simulink model "HANcoder_E407_GTSync_v5"  (R2018b)
settings: Solver=FixedStepDiscrete  StartTime=0.0  StopTime=1  FixedStep=0.01  RelTol=1e-3
PreLoadFcn:
  | librarySetup
  | eval([bdroot,'_startup']) %Calling [modelName]_startup.m
values from neighbouring files (symbols this model uses):
  basic_cycle_duration = TM_Reset_Board + COMP_duration    (= 170)    [HANcoder_E407_GTSync_v5_startup.m]
  comm_delay_estimation1 = round(comm_delay_measured*hardware_granularity/frequency_IRQ)    [HANcoder_E407_GTSync_v5_startup.m]
  comm_delay_estimation2 = round(comm_delay_measured*hardware_granularity/frequency_IRQ)    [HANcoder_E407_GTSync_v5_startup.m]
  COMM_Period = 25    [HANcoder_E407_GTSync_v5_startup.m]
  COMM_Phase1 = floor(COMM_Period/5)    [HANcoder_E407_GTSync_v5_startup.m]
  COMM_Phase2 = floor(4*COMM_Period/5)    [HANcoder_E407_GTSync_v5_startup.m]
  frequency_IRQ = 100    [HANcoder_E407_GTSync_v5_startup.m]
  HANtuneOverride = Simulink.Parameter    [HANcoder_E407_GTSync_v5_startup.m]
  idle_time_init = basic_cycle_duration*matrix_rows    (= 340)    [HANcoder_E407_GTSync_v5_startup.m]
  LED_ticks_toggle = 10000    [HANcoder_E407_GTSync_v5_startup.m]
  Master_Role = 1    [HANcoder_E407_GTSync_v5_startup.m]
  matrix_rows = 2    [HANcoder_E407_GTSync_v5_startup.m]
  MEX_Flag = 0    [HANcoder_E407_GTSync_v5_startup.m]
  Slave_Role = 2    [HANcoder_E407_GTSync_v5_startup.m]
  Sync_ID = 1    [HANcoder_E407_GTSync_v5_startup.m]
  TM_Check_Sync = TM_COMM_Sync   + COMM_duration    (= 30)    [HANcoder_E407_GTSync_v5_startup.m]
  TM_Check_TOuts = TM_Count_Vote3 + COMP_duration    (= 150)    [HANcoder_E407_GTSync_v5_startup.m]
  TM_Check_Vote1 = TM_COMM_Vote1  + COMM_duration    (= 70)    [HANcoder_E407_GTSync_v5_startup.m]
  TM_Check_Vote2 = TM_COMM_Vote2  + COMM_duration    (= 105)    [HANcoder_E407_GTSync_v5_startup.m]
  TM_Check_Vote3 = TM_COMM_Vote3  + COMM_duration    (= 140)    [HANcoder_E407_GTSync_v5_startup.m]
  TM_COMM_Sync = basic_cycle_start    (= 5)    [HANcoder_E407_GTSync_v5_startup.m]
  TM_COMM_Vote1 = TM_Vote_Dec    + COMP_duration    (= 45)    [HANcoder_E407_GTSync_v5_startup.m]
  TM_COMM_Vote2 = TM_Count_Vote1 + COMP_duration    (= 80)    [HANcoder_E407_GTSync_v5_startup.m]
  TM_COMM_Vote3 = TM_Count_Vote2 + COMP_duration    (= 115)    [HANcoder_E407_GTSync_v5_startup.m]
  TM_Count_Vote1 = TM_Check_Vote1 + COMP_duration    (= 75)    [HANcoder_E407_GTSync_v5_startup.m]
  TM_Count_Vote2 = TM_Check_Vote2 + COMP_duration    (= 110)    [HANcoder_E407_GTSync_v5_startup.m]
  TM_Count_Vote3 = TM_Check_Vote3 + COMP_duration    (= 145)    [HANcoder_E407_GTSync_v5_startup.m]
  TM_New_Master = TM_Check_TOuts + COMP_duration    (= 155)    [HANcoder_E407_GTSync_v5_startup.m]
  TM_Reset_Board = TM_Reset_Var   + COMP_duration    (= 165)    [HANcoder_E407_GTSync_v5_startup.m]
  TM_Reset_Var = TM_New_Master  + COMP_duration    (= 160)    [HANcoder_E407_GTSync_v5_startup.m]
  TM_Update_LT = TM_Check_Sync  + COMP_duration    (= 35)    [HANcoder_E407_GTSync_v5_startup.m]
  TM_Vote_Dec = TM_Update_LT   + COMP_duration    (= 40)    [HANcoder_E407_GTSync_v5_startup.m]
  Toggle_Flag = 1    [HANcoder_E407_GTSync_v5_startup.m]
  Vote1_ID = 12    [HANcoder_E407_GTSync_v5_startup.m]
  Vote2_ID = 22    [HANcoder_E407_GTSync_v5_startup.m]
  Vote3_ID = 32    [HANcoder_E407_GTSync_v5_startup.m]
undefined symbols (not defined in the file or in its folder): A0, A1, A2, A3, CON2
libraries: HANcoder_STM32_Target x25, hdlsllib x21, simulink x3, simulink_extras x1
(part 2 of 7)

== system HANcoder_E407_GTSync_v5/HANcoder STM32 Target - E407-STM32 algorithm/Global Ticks Increment/If Action Subsystem ==
  note: CAN ID Init
  Action Port : ActionPort  ActionType=then
  Add : Sum  Inputs=++++
  Constant : Constant
  Constant1 : Constant  Value=2
  Constant2 : Constant  Value=4
  Constant3 : Constant  Value=8
  Digital Input : HANcoder_STM32_Target/STM32-E407/Digital Inputs/Digital Input  Tag=HANcoder_TARGET_STM32_E407  pinID=CON3 - D2 - 5V Tolerant  config=Pulldown  tsamp=-1
      settings: SourceProductName=HANcoder STM32 Target
  Digital Input1 : HANcoder_STM32_Target/STM32-E407/Digital Inputs/Digital Input  Tag=HANcoder_TARGET_STM32_E407  pinID=CON3 - D3 - 5V Tolerant  config=Pulldown  tsamp=-1
      settings: SourceProductName=HANcoder STM32 Target
  Digital Input2 : HANcoder_STM32_Target/STM32-E407/Digital Inputs/Digital Input  Tag=HANcoder_TARGET_STM32_E407  pinID=CON3 - D4 - 5V Tolerant  config=Pulldown  tsamp=-1
      settings: SourceProductName=HANcoder STM32 Target
  Digital Input3 : HANcoder_STM32_Target/STM32-E407/Digital Inputs/Digital Input  Tag=HANcoder_TARGET_STM32_E407  pinID=CON3 - D5 - 5V Tolerant  config=Pulldown  tsamp=-1
      settings: SourceProductName=HANcoder STM32 Target
  Multiply{,1..3} (4 alike) : Product
  Out1 : Outport
  wires:
  Constant1/1 -> Multiply1/1
  Add/1 -> Out1/1
  Constant3/1 -> Multiply3/1
  Constant2/1 -> Multiply2/1
  Multiply2/1 -> Add/3
  Digital Input3/1 -> Multiply3/2
  Digital Input1/1 -> Multiply1/2
  Multiply3/1 -> Add/4
  Multiply1/1 -> Add/2
  Digital Input2/1 -> Multiply2/2
  Multiply/1 -> Add/1
  Digital Input/1 -> Multiply/2
  Constant/1 -> Multiply/1

== system HANcoder_E407_GTSync_v5/HANcoder STM32 Target - E407-STM32 algorithm/Global Ticks Increment/Initialize Clock Schedule ==
  Enable : EnablePort
  Constant : Constant  OutDataTypeStr=uint16
  Constant1 : Constant  Value=3  OutDataTypeStr=uint8
  Constant2 : Constant
  Data Store Write : DataStoreWrite  DataStoreName=init_clock
  Schedule Compare Event1 : HANcoder_STM32_Target/STM32-E407/Timer Outputs/Schedule Compare Event  Tag=HANcoder_TARGET_STM32_E407  pin=TIM4 - CON PD - 15 - 5V Tolerant  tsamp=-1
      settings: SourceProductName=HANcoder STM32 Target
  wires:
  Constant/1 -> Schedule Compare Event1/1
  Constant1/1 -> Schedule Compare Event1/2
  Constant2/1 -> Data Store Write/1

== system HANcoder_E407_GTSync_v5/HANcoder STM32 Target - E407-STM32 algorithm/Global Ticks Increment/Local Time generation ==
  note: Reschedule IRQ activation
  Clock_State : Inport
  function : TriggerPort  TriggerType=function-call  VariantControl=Variant
  Chart : Stateflow chart  TreatAsAtomicUnit=on
  Constant : Constant  Value=frequency_IRQ  OutDataTypeStr=uint16
  Constant1 : Constant  Value=3  OutDataTypeStr=uint8
  Constant2 : Constant  OutDataTypeStr=uint16
  Data Store Read : DataStoreRead  DataStoreName=Local_Ticks
  Data Store Read1 : DataStoreRead  DataStoreName=Local_Ticks
  Data Store Write : DataStoreWrite  DataStoreName=Local_Ticks
  Get Last Event Counter1 : HANcoder_STM32_Target/STM32-E407/Timer Outputs/Get Last Event Counter  Tag=HANcoder_TARGET_STM32_E407  pin=TIM4 - CON PD - 15 - 5V Tolerant  tsamp=-1
      settings: SourceProductName=HANcoder STM32 Target
  Schedule Compare Event : HANcoder_STM32_Target/STM32-E407/Timer Outputs/Schedule Compare Event  Tag=HANcoder_TARGET_STM32_E407  pin=TIM4 - CON PD - 15 - 5V Tolerant  tsamp=-1
      settings: SourceProductName=HANcoder STM32 Target
  Sum : Sum
  Sum1 : Sum
  Switch : Switch  Criteria=u2 > Threshold
  activate_CAN_management : Outport
  wires:
  Get Last Event Counter1/1 -> Sum/1
  Constant/1 -> Sum/2
  Sum/1 -> Schedule Compare Event/1
  Constant1/1 -> Schedule Compare Event/2
  Data Store Read1/1 -> Switch/3
  Data Store Read/1 -> Sum1/1
  Constant2/1 -> Sum1/2
  Clock_State/1 -> Chart/1(Condition), Switch/2
  Switch/1 -> Data Store Write/1  "local_ticks_interrupt"
  Sum1/1 -> Switch/1
  Chart/1(Trigger_Signal()) -> activate_CAN_management/1

== system HANcoder_E407_GTSync_v5/HANcoder STM32 Target - E407-STM32 algorithm/Global Ticks Increment/Measure EXecution time ==
  note: Measured Execution Time
  Trigger : TriggerPort  TriggerType=function-call  VariantControl=Variant
  Constant1 : Constant  Priority=1  Value=MEX_Flag
  DEBUG - Toggle digital pin A3 : Subsystem  Priority=3
  Data Store Memory4 : DataStoreMemory  DataStoreName=A3_Pin_State  ReadBeforeWriteMsg=warning  WriteAfterWriteMsg=warning  WriteAfterReadMsg=warning  ShowAdditionalParam=off  OutDataTypeStr=boolean
  wires:
  Constant1/1 -> DEBUG - Toggle digital pin A3/Enable

== system HANcoder_E407_GTSync_v5/HANcoder STM32 Target - E407-STM32 algorithm/Global Ticks Increment/Output Compare Init2 ==
  S-Function : S-Function  FunctionName=sfcn_timeout_init  SFunctionDeploymentMode=off  EnableBusSupport=off
  Term1 : Terminator
  wires:
  S-Function/1 -> Term1/1

== system HANcoder_E407_GTSync_v5/HANcoder STM32 Target - E407-STM32 algorithm/Operation Mode/Flip Flop T ==
  T : Inport  OutDataTypeStr=boolean
  Clk : Inport  Port=2  OutDataTypeStr=boolean
  J-K Flip-Flop : simulink_extras/Flip Flops/J-K Flip-Flop  initial_condition=0
      settings: SourceProductName=Simulink
  Terminator : Terminator
  Q : Outport  OutDataTypeStr=boolean
  wires:
  J-K Flip-Flop/2 -> Terminator/1
  T/1 -> J-K Flip-Flop/3, J-K Flip-Flop/1
  J-K Flip-Flop/1 -> Q/1
  Clk/1 -> J-K Flip-Flop/2

== system HANcoder_E407_GTSync_v5/HANcoder STM32 Target - E407-STM32 algorithm/Global Ticks Increment/CAN Management/Basic Cycle Increment ==
  note: Local Time Reset
  note: Basic cycle counter
  Enable : EnablePort
  Add : Sum
  Add1 : Sum  Inputs=+-
  Constant : Constant  Value=matrix_rows
  Data Store Read4 : DataStoreRead  DataStoreName=basic_cycle_count
  Data Store Read5 : DataStoreRead  DataStoreName=basic_cycle_count
  Data Store Write : DataStoreWrite  DataStoreName=Local_Ticks
  Data Store Write3 : DataStoreWrite  DataStoreName=basic_cycle_count
  Decrement : Constant  OutDataTypeStr=uint8
  Increment : Constant  OutDataTypeStr=uint8
  LessThanOrEqual : RelationalOperator  Operator=<  OutDataTypeStr=boolean  RndMeth=Simplest
  Reset : Constant  Value=0  OutDataTypeStr=uint16
  Switch : Switch  Criteria=u2 > Threshold
  wires:
  Switch/1 -> Data Store Write3/1  "bc"
  Data Store Read5/1 -> LessThanOrEqual/1
  Add/1 -> Switch/1
  Increment/1 -> Add/2
  Data Store Read4/1 -> Add/1
  LessThanOrEqual/1 -> Switch/2
  Constant/1 -> Add1/1
  Reset/1 -> Switch/3, Data Store Write/1
  Decrement/1 -> Add1/2
  Add1/1 -> LessThanOrEqual/2

== system HANcoder_E407_GTSync_v5/HANcoder STM32 Target - E407-STM32 algorithm/Global Ticks Increment/CAN Management/DEBUG - Toggle digital pin A0 ==
  note: Change pin state
  note: Reset condition
  note: Toggle pin data stored
  Enable : EnablePort
  Constant : Constant  OutDataTypeStr=boolean
  Constant1 : Constant  Value=0  OutDataTypeStr=boolean
  Constant2 : Constant  Value=0  OutDataTypeStr=boolean
  Data Store Read : DataStoreRead  DataStoreName=A0_Pin_State
  Data Store Read1 : DataStoreRead  DataStoreName=A0_Pin_State
  Data Store Write : DataStoreWrite  DataStoreName=Toggle_Pin_A0
  Data Store Write1 : DataStoreWrite  DataStoreName=A0_Pin_State
  Digital Output : HANcoder_STM32_Target/STM32-E407/Digital Outputs/Digital Output  Tag=HANcoder_TARGET_STM32_E407  pinID=CON2 - A0  config=Open drain  tsamp=-1
      settings: SourceProductName=HANcoder STM32 Target
  Switch : Switch  Criteria=u2 > Threshold
  wires:
  Switch/1 -> Data Store Write1/1
  Data Store Read/1 -> Switch/2
  Constant/1 -> Switch/3
  Constant1/1 -> Switch/1
  Constant2/1 -> Data Store Write/1
  Data Store Read1/1 -> Digital Output/1

== system HANcoder_E407_GTSync_v5/HANcoder STM32 Target - E407-STM32 algorithm/Global Ticks Increment/CAN Management/DEBUG - Toggle digital pin A1 ==
  note: Toggle pin data stored
  note: Reset condition
  note: Change pin state
  Enable : EnablePort
  Constant : Constant  OutDataTypeStr=boolean
  Constant1 : Constant  Value=0  OutDataTypeStr=boolean
  Constant2 : Constant  Value=0  OutDataTypeStr=boolean
  Data Store Read : DataStoreRead  DataStoreName=A1_Pin_State
  Data Store Read1 : DataStoreRead  DataStoreName=A1_Pin_State
  Data Store Write : DataStoreWrite  DataStoreName=Toggle_Pin_A1
  Data Store Write1 : DataStoreWrite  DataStoreName=A1_Pin_State
  Digital Output : HANcoder_STM32_Target/STM32-E407/Digital Outputs/Digital Output  Tag=HANcoder_TARGET_STM32_E407  pinID=CON2 - A1  config=Open drain  tsamp=-1
      settings: SourceProductName=HANcoder STM32 Target
  Switch : Switch  Criteria=u2 > Threshold
  wires:
  Data Store Read1/1 -> Digital Output/1
  Constant2/1 -> Data Store Write/1
  Constant1/1 -> Switch/1
  Constant/1 -> Switch/3
  Data Store Read/1 -> Switch/2
  Switch/1 -> Data Store Write1/1

== system HANcoder_E407_GTSync_v5/HANcoder STM32 Target - E407-STM32 algorithm/Global Ticks Increment/CAN Management/DEBUG - Toggle digital pin A2 ==
  note: Toggle pin data stored
  note: Change pin state
  Enable : EnablePort
  Constant : Constant  OutDataTypeStr=boolean
  Constant1 : Constant  Value=0  OutDataTypeStr=boolean
  Data Store Read : DataStoreRead  DataStoreName=A2_Pin_State
  Data Store Read1 : DataStoreRead  DataStoreName=A2_Pin_State
  Data Store Write1 : DataStoreWrite  DataStoreName=A2_Pin_State
  Digital Output : HANcoder_STM32_Target/STM32-E407/Digital Outputs/Digital Output  Tag=HANcoder_TARGET_STM32_E407  pinID=CON2 - A2  config=Open drain  tsamp=-1
      settings: SourceProductName=HANcoder STM32 Target
  Switch : Switch  Criteria=u2 > Threshold
  wires:
  Data Store Read1/1 -> Digital Output/1
  Constant1/1 -> Switch/1
  Constant/1 -> Switch/3
  Data Store Read/1 -> Switch/2
  Switch/1 -> Data Store Write1/1

== system HANcoder_E407_GTSync_v5/HANcoder STM32 Target - E407-STM32 algorithm/Global Ticks Increment/CAN Management/Initialization ==
  Enable : EnablePort  PropagateVarSize=During execution
  AND : Logic  IconShape=distinctive  AllPortsSameDT=off  OutDataTypeStr=boolean
  Board nr1 : Constant
  Constant : Constant  Value=idle_time_init
  Data Store Memory : DataStoreMemory  DataStoreName=Initialization_Timeout  ReadBeforeWriteMsg=warning  WriteAfterWriteMsg=warning  WriteAfterReadMsg=warning  ShowAdditionalParam=off  OutDataTypeStr=boolean
  Data Store Memory1 : DataStoreMemory  DataStoreName=Delay_Counter  ReadBeforeWriteMsg=warning  WriteAfterWriteMsg=warning  WriteAfterReadMsg=warning  ShowAdditionalParam=off  OutDataTypeStr=double
  Data Store Read : DataStoreRead  DataStoreName=New_Msg_Ready_CAN1
  Data Store Read1 : DataStoreRead  DataStoreName=Initialization_Timeout
  Data Store Read2 : DataStoreRead  DataStoreName=New_Msg_Ready_CAN2
  Data Store Read4 : DataStoreRead  DataStoreName=Board_ID
  Data Store Write : DataStoreWrite  DataStoreName=Initialization_Timeout
  Data Store Write1 : DataStoreWrite  DataStoreName=Initialization_flag
  Delay : Subsystem
  Equal : RelationalOperator  Operator===  OutDataTypeStr=boolean  RndMeth=Simplest
  NOT : Logic  Operator=NOT  IconShape=distinctive  AllPortsSameDT=off  OutDataTypeStr=boolean
  OR : Logic  Operator=OR  IconShape=distinctive  AllPortsSameDT=off  OutDataTypeStr=boolean
  OR1 : Logic  Operator=OR  IconShape=distinctive  AllPortsSameDT=off  OutDataTypeStr=boolean
  RoleID and Global Time init : Subsystem  TreatAsAtomicUnit=on
  wires:
  Delay/1(Output) -> Data Store Write/1
  Constant/1 -> Delay/1(Input)
  NOT/1 -> Data Store Write1/1
  RoleID and Global Time init/1(Finish Initialization) -> NOT/1
  OR/1 -> RoleID and Global Time init/Enable
  Data Store Read1/1 -> AND/2, RoleID and Global Time init/1(Timeout Initialization)
  OR1/1 -> OR/2, RoleID and Global Time init/2(Reference message received)
  Data Store Read4/1 -> Equal/1
  Board nr1/1 -> Equal/2
  Equal/1 -> AND/1
  AND/1 -> OR/1
  Data Store Read/1 -> OR1/1
  Data Store Read2/1 -> OR1/2

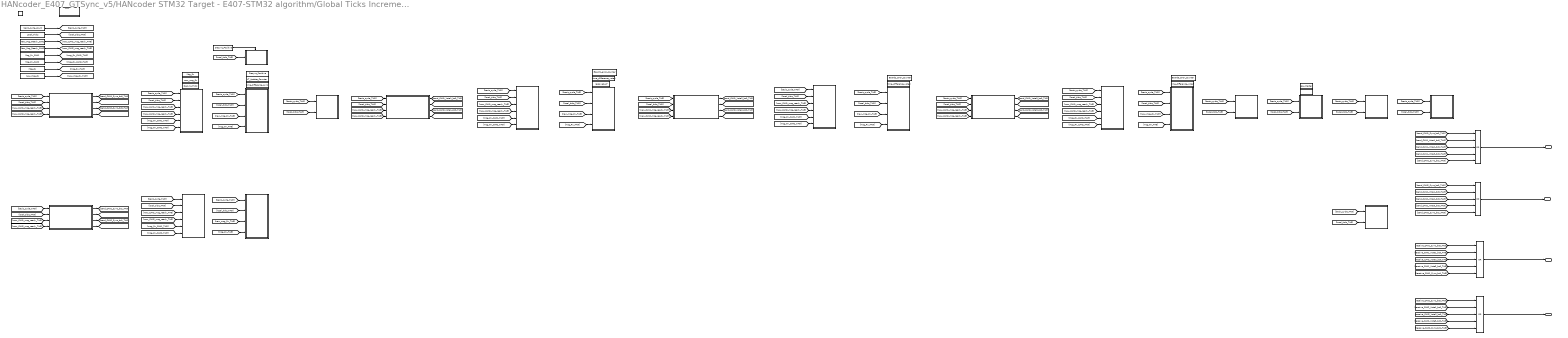
== system HANcoder_E407_GTSync_v5/HANcoder STM32 Target - E407-STM32 algorithm/Global Ticks Increment/CAN Management/Matrix Cycle Manager ==
  note: Receive message condition
      | Sync Msg: Not Master and TM0
      | Vote Msg: Not # Node at TM#
  note: Shortcut Tags
  note: Output Send_Message
      | Send: 1
      | Do not send: 0
  note: Send message condition
      | Sync Msg: Master and TM0
      | Vote Msg: Node# and TM#
  note: Output Receive_Message
      | Receive: 1
      | Do not receive: 0
  note: Receive message condition
      | Sync Msg: Not Master and TM0
      | Vote Msg: Not # Node at TM#
  note: Output Receive_Message
      | Receive: 1
      | Do not receive: 0
  note: Send message condition
      | Sync Msg: Master and TM0
      | Vote Msg: Node# and TM#
  note: Output Send_Message
      | Send: 1
      | Do not send: 0
  Enable : EnablePort  PropagateVarSize=During execution
  COMM Task - Sync BC0 : Subsystem
  COMM Task - Sync BC1 : Subsystem
  COMM Task - Vote1 : Subsystem
  COMM Task - Vote2 : Subsystem
  COMM Task - Vote3 : Subsystem
  COMP Task - Check Timeouts : Subsystem
  COMP Task - New Master : Subsystem
  COMP Task - Reset Board : Subsystem
  COMP Task - Reset Variables BC0 : Subsystem
  COMP Task - Reset Variables BC1 : Subsystem
  COMP Task - Rx_Sync_Check : Subsystem
  COMP Task - Rx_Sync_Check - bc1 : Subsystem
  COMP Task - Rx_Vote1_Check : Subsystem
  COMP Task - Rx_Vote2_Check : Subsystem
  COMP Task - Rx_Vote3_Check : Subsystem
  COMP Task - Update LT : Subsystem
  COMP Task - Update LT - bc1 : Subsystem
  COMP Task - Vote Decision : Subsystem
  COMP Task - Vote1 Count : Subsystem
  COMP Task - Vote2 Count : Subsystem
  COMP Task - Vote3 Count : Subsystem
  Data Store Memory : DataStoreMemory  DataStoreName=time_difference_sync  ReadBeforeWriteMsg=warning  WriteAfterWriteMsg=warning  WriteAfterReadMsg=warning  ShowAdditionalParam=off
  Data Store Memory1 : DataStoreMemory  DataStoreName=Board1_error_counter  ReadBeforeWriteMsg=warning  WriteAfterWriteMsg=warning  WriteAfterReadMsg=warning  ShowAdditionalParam=off  OutMin=0  OutMax=4294967294  OutDataTypeStr=double
  Data Store Memory10 : DataStoreMemory  DataStoreName=New_Master  ReadBeforeWriteMsg=warning  WriteAfterWriteMsg=warning  WriteAfterReadMsg=warning  ShowAdditionalParam=off  OutDataTypeStr=boolean
  Data Store Memory11 : DataStoreMemory  DataStoreName=Msg_Rx  ReadBeforeWriteMsg=warning  WriteAfterWriteMsg=warning  WriteAfterReadMsg=warning  ShowAdditionalParam=off  OutDataTypeStr=Bus: demux_msg_buffer_type
  Data Store Memory12 : DataStoreMemory  DataStoreName=LT_Update_Counter  ReadBeforeWriteMsg=warning  WriteAfterWriteMsg=warning  WriteAfterReadMsg=warning  ShowAdditionalParam=off
  Data Store Memory13 : DataStoreMemory  DataStoreName=Desync_Ticks  ReadBeforeWriteMsg=warning  WriteAfterWriteMsg=warning  WriteAfterReadMsg=warning  ShowAdditionalParam=off  OutDataTypeStr=double
  Data Store Memory14 : DataStoreMemory  DataStoreName=Desync_Positive  ReadBeforeWriteMsg=warning  WriteAfterWriteMsg=warning  WriteAfterReadMsg=warning  ShowAdditionalParam=off  OutDataTypeStr=boolean
  Data Store Memory2 : DataStoreMemory  DataStoreName=Board2_error_counter  ReadBeforeWriteMsg=warning  WriteAfterWriteMsg=warning  WriteAfterReadMsg=warning  ShowAdditionalParam=off  OutMin=0  OutMax=4294967294  OutDataTypeStr=double
  Data Store Memory3 : DataStoreMemory  DataStoreName=Board3_error_counter  ReadBeforeWriteMsg=warning  WriteAfterWriteMsg=warning  WriteAfterReadMsg=warning  ShowAdditionalParam=off  OutMin=0  OutMax=4294967294  OutDataTypeStr=double
  Data Store Memory4 : DataStoreMemory  DataStoreName=time_difference_vote1  ReadBeforeWriteMsg=warning  WriteAfterWriteMsg=warning  WriteAfterReadMsg=warning  ShowAdditionalParam=off
  Data Store Memory5 : DataStoreMemory  DataStoreName=time_difference_vote2  ReadBeforeWriteMsg=warning  WriteAfterWriteMsg=warning  WriteAfterReadMsg=warning  ShowAdditionalParam=off
  Data Store Memory6 : DataStoreMemory  DataStoreName=time_difference_vote3  ReadBeforeWriteMsg=warning  WriteAfterWriteMsg=warning  WriteAfterReadMsg=warning  ShowAdditionalParam=off
  Data Store Memory7 : DataStoreMemory  DataStoreName=Reset_Board  ReadBeforeWriteMsg=warning  WriteAfterWriteMsg=warning  WriteAfterReadMsg=warning  ShowAdditionalParam=off  OutDataTypeStr=boolean
  Data Store Memory8 : DataStoreMemory  DataStoreName=new_msg_Rx  ReadBeforeWriteMsg=warning  WriteAfterWriteMsg=warning  WriteAfterReadMsg=warning  ShowAdditionalParam=off
  Data Store Memory9 : DataStoreMemory  DataStoreName=received_LT  ReadBeforeWriteMsg=warning  WriteAfterWriteMsg=warning  WriteAfterReadMsg=warning  ShowAdditionalParam=off  OutDataTypeStr=Bus: received_vote_local_time
  Data Store Read : DataStoreRead  DataStoreName=Msg_Rx_CAN1
  Data Store Read1 : DataStoreRead  DataStoreName=New_Msg_Ready_CAN1
  Data Store Read10 : DataStoreRead  DataStoreName=basic_cycle_count
  Data Store Read2 : DataStoreRead  DataStoreName=New_Msg_Ready_CAN2
  Data Store Read3 : DataStoreRead  DataStoreName=Msg_Rx_CAN2
  Data Store Read4 : DataStoreRead  DataStoreName=Msg_Rx
  Data Store Read5 : DataStoreRead  DataStoreName=new_msg_Rx
  Data Store Read6 : DataStoreRead  DataStoreName=Desync_Positive
  Data Store Read9 : DataStoreRead  DataStoreName=Local_Ticks
  LT_Update Desync_Positive : Subsystem  Priority=100  TreatAsAtomicUnit=on
  Matrix_Cycle_Observation_DEBUG : Subsystem
  OR{1..4} (4 alike) : Logic  Operator=OR  Inputs=5  IconShape=distinctive  AllPortsSameDT=off  OutDataTypeStr=boolean
  Send_Message_CAN1 : Outport
  Send_Message_CAN2 : Outport  Port=2
  Receive_Message_CAN1 : Outport  Port=3
  Receive_Message_CAN2 : Outport  Port=4
  wires:
  Data Store Read10/1 -> [basic_cycle_TAG]
  OR1/1 -> Send_Message_CAN1/1
  Data Store Read9/1 -> [local_ticks_TAG]  "local_time_s"
  [basic_cycle_TAG] -> COMM Task - Sync BC0/1(basic_cycle)
  [local_ticks_TAG] -> COMM Task - Sync BC0/2(local_time)
  [basic_cycle_TAG] -> COMP Task - Update LT/1(basic cycle)
  [local_ticks_TAG] -> COMP Task - Update LT/2(local time)
  COMM Task - Sync BC0/1(send_new_msg_CAN1) -> [send_CAN1_Sync_bc0_TAG]
  COMM Task - Sync BC0/2(receive new msg CAN1) -> [receive_CAN1_Sync_bc0_TAG]
  [local_ticks_TAG] -> COMP Task - Vote Decision/2(local time)
  [basic_cycle_TAG] -> COMP Task - Vote Decision/1(basic cycle)
  COMM Task - Vote1/2(receive_new_msg_CAN1) -> [receive_CAN1_Vote1_bc0_TAG]
  COMM Task - Vote1/1(send_new_msg_CAN1) -> [send_CAN1_Vote1_bc0_TAG]
  [local_ticks_TAG] -> COMM Task - Vote1/2(local_time)
  [basic_cycle_TAG] -> COMM Task - Vote1/1(basic_cycle)
  [local_ticks_TAG] -> COMP Task - Vote1 Count/2(local time)
  [basic_cycle_TAG] -> COMP Task - Vote1 Count/1(basic cycle)
  [basic_cycle_TAG] -> COMM Task - Vote2/1(basic_cycle)
  [local_ticks_TAG] -> COMM Task - Vote2/2(local_time)
  COMM Task - Vote2/1(send_new_msg_CAN1) -> [send_CAN1_Vote2_bc0_TAG]
  COMM Task - Vote2/2(receive_new_msg_CAN1) -> [receive_CAN1_Vote2_bc0_TAG]
  COMM Task - Vote3/2(receive_new_msg_CAN1) -> [receive_CAN1_Vote3_bc0_TAG]
  COMM Task - Vote3/1(send_new_msg_CAN1) -> [send_CAN1_Vote3_bc0_TAG]
  [local_ticks_TAG] -> COMM Task - Vote3/2(local_time)
  [basic_cycle_TAG] -> COMM Task - Vote3/1(basic_cycle)
  [basic_cycle_TAG] -> COMP Task - Vote2 Count/1(basic cycle)
  [local_ticks_TAG] -> COMP Task - Vote2 Count/2(local time)
  [local_ticks_TAG] -> COMP Task - Vote3 Count/2(local time)
  [basic_cycle_TAG] -> COMP Task - Vote3 Count/1(basic cycle)
  [basic_cycle_TAG] -> COMP Task - Check Timeouts/1(basic cycle)
  [local_ticks_TAG] -> COMP Task - Check Timeouts/2(local time)
  [local_ticks_TAG] -> COMP Task - New Master/2(local time)
  [basic_cycle_TAG] -> COMP Task - New Master/1(basic cycle)
  [basic_cycle_TAG] -> COMP Task - Reset Variables BC0/1(basic cycle)
  [local_ticks_TAG] -> COMP Task - Reset Variables BC0/2(local time)
  [local_ticks_TAG] -> COMP Task - Reset Variables BC1/2(local time)
  [basic_cycle_TAG] -> COMP Task - Reset Variables BC1/1(basic cycle)
  [send_CAN1_Sync_bc0_TAG] -> OR1/1
  [send_CAN1_Vote1_bc0_TAG] -> OR1/2
  [send_CAN1_Vote2_bc0_TAG] -> OR1/3
  [send_CAN1_Vote3_bc0_TAG] -> OR1/4
  [receive_CAN1_Vote3_bc0_TAG] -> OR2/4
  [receive_CAN1_Vote2_bc0_TAG] -> OR2/3
  [receive_CAN1_Vote1_bc0_TAG] -> OR2/2
  [receive_CAN1_Sync_bc0_TAG] -> OR2/1
  [local_ticks_TAG] -> COMP Task - Reset Board/2(local time)
  [basic_cycle_TAG] -> COMP Task - Reset Board/1(basic cycle)
  OR2/1 -> Receive_Message_CAN1/1
  [send_CAN1_Sync_bc1_TAG] -> OR1/5
  [receive_CAN1_Sync_bc1_TAG] -> OR2/5
  [basic_cycle_TAG] -> COMP Task - Update LT - bc1/1(basic cycle)
  Data Store Read1/1 -> [new_CAN1_msg_ready_TAG]
  [new_CAN1_msg_ready_TAG] -> COMM Task - Sync BC0/3(new_message_CAN1)
  [new_CAN1_msg_ready_TAG] -> COMM Task - Vote1/3(new_message_CAN1)
  [new_msg_Rx_TAG] -> COMP Task - Vote1 Count/3(new_message)
  [new_CAN1_msg_ready_TAG] -> COMM Task - Vote2/3(new_message_CAN1)
  [new_msg_Rx_TAG] -> COMP Task - Vote2 Count/3(new_message)
  [new_CAN1_msg_ready_TAG] -> COMM Task - Vote3/3(new_message_CAN1)
  [new_msg_Rx_TAG] -> COMP Task - Vote3 Count/3(new_message)
  COMM Task - Sync BC0/3(send_new_msg_CAN2) -> [send_CAN2_Sync_bc0_TAG]
  COMM Task - Sync BC0/4(receive_new_msg_CAN2) -> [receive_CAN2_Sync_bc0_TAG]
  [new_CAN2_msg_ready_TAG] -> COMM Task - Sync BC0/4(new_message_CAN2)
  Data Store Read2/1 -> [new_CAN2_msg_ready_TAG]
  [new_CAN2_msg_ready_TAG] -> COMM Task - Vote1/4(new_message_CAN2)
  COMM Task - Vote1/3(send_new_msg_CAN2) -> [send_CAN2_Vote1_bc0_TAG]
  COMM Task - Vote1/4(receive_new_msg_CAN2) -> [receive_CAN2_Vote1_bc0_TAG]
  [new_CAN2_msg_ready_TAG] -> COMM Task - Vote2/4(new_message_CAN2)
  COMM Task - Vote2/3(send_new_msg_CAN2) -> [send_CAN2_Vote2_bc0_TAG]
  COMM Task - Vote2/4(receive_new_msg_CAN2) -> [receive_CAN2_Vote2_bc0_TAG]
  [new_CAN2_msg_ready_TAG] -> COMM Task - Vote3/4(new_message_CAN2)
  COMM Task - Vote3/3(send_new_msg_CAN2) -> [send_CAN2_Vote3_bc0_TAG]
  COMM Task - Vote3/4(receive_new_msg_CAN2) -> [receive_CAN2_Vote3_bc0_TAG]
  [receive_CAN2_Sync_bc1_TAG] -> OR3/5
  OR3/1 -> Receive_Message_CAN2/1
  [receive_CAN2_Sync_bc0_TAG] -> OR3/1
  [receive_CAN2_Vote1_bc0_TAG] -> OR3/2
  [receive_CAN2_Vote2_bc0_TAG] -> OR3/3
  [receive_CAN2_Vote3_bc0_TAG] -> OR3/4
  [send_CAN2_Sync_bc1_TAG] -> OR4/5
  [send_CAN2_Vote3_bc0_TAG] -> OR4/4
  [send_CAN2_Vote2_bc0_TAG] -> OR4/3
  [send_CAN2_Vote1_bc0_TAG] -> OR4/2
  [send_CAN2_Sync_bc0_TAG] -> OR4/1
  OR4/1 -> Send_Message_CAN2/1
  [new_CAN1_msg_ready_TAG] -> COMP Task - Rx_Sync_Check/3(new_CAN1_msg)
  [new_CAN2_msg_ready_TAG] -> COMP Task - Rx_Sync_Check/4(new_CAN2_msg)
  [local_ticks_TAG] -> COMP Task - Rx_Sync_Check/2(local_time)
  [basic_cycle_TAG] -> COMP Task - Rx_Sync_Check/1(basic_cycle)
  Data Store Read/1 -> [msg_Rx_CAN1_TAG]
  Data Store Read3/1 -> [msg_Rx_CAN2_TAG]
  [msg_Rx_CAN1_TAG] -> COMP Task - Rx_Sync_Check/5(Rx_msg_CAN1)
  [msg_Rx_CAN2_TAG] -> COMP Task - Rx_Sync_Check/6(Rx_msg_CAN2)
  Data Store Read4/1 -> [msg_Rx_TAG]
  Data Store Read5/1 -> [new_msg_Rx_TAG]
  [new_msg_Rx_TAG] -> COMP Task - Update LT/3(new_message)
  [msg_Rx_TAG] -> COMP Task - Update LT/4(Rx_msg)
  [msg_Rx_CAN2_TAG] -> COMP Task - Rx_Vote1_Check/6(Rx_msg_CAN2)
  [msg_Rx_CAN1_TAG] -> COMP Task - Rx_Vote1_Check/5(Rx_msg_CAN1)
  [basic_cycle_TAG] -> COMP Task - Rx_Vote1_Check/1(basic_cycle)
  [local_ticks_TAG] -> COMP Task - Rx_Vote1_Check/2(local_time)
  [new_CAN2_msg_ready_TAG] -> COMP Task - Rx_Vote1_Check/4(new_CAN2_msg)
  [new_CAN1_msg_ready_TAG] -> COMP Task - Rx_Vote1_Check/3(new_CAN1_msg)
  [new_CAN1_msg_ready_TAG] -> COMP Task - Rx_Vote2_Check/3(new_CAN1_msg)
  [new_CAN2_msg_ready_TAG] -> COMP Task - Rx_Vote2_Check/4(new_CAN2_msg)
  [local_ticks_TAG] -> COMP Task - Rx_Vote2_Check/2(local_time)
  [basic_cycle_TAG] -> COMP Task - Rx_Vote2_Check/1(basic_cycle)
  [msg_Rx_CAN1_TAG] -> COMP Task - Rx_Vote2_Check/5(Rx_msg_CAN1)
  [msg_Rx_CAN2_TAG] -> COMP Task - Rx_Vote2_Check/6(Rx_msg_CAN2)
  [msg_Rx_CAN2_TAG] -> COMP Task - Rx_Vote3_Check/6(Rx_msg_CAN2)
  [msg_Rx_CAN1_TAG] -> COMP Task - Rx_Vote3_Check/5(Rx_msg_CAN1)
  [basic_cycle_TAG] -> COMP Task - Rx_Vote3_Check/1(basic_cycle)
  [local_ticks_TAG] -> COMP Task - Rx_Vote3_Check/2(local_time)
  [new_CAN2_msg_ready_TAG] -> COMP Task - Rx_Vote3_Check/4(new_CAN2_msg)
  [new_CAN1_msg_ready_TAG] -> COMP Task - Rx_Vote3_Check/3(new_CAN1_msg)
  COMM Task - Sync BC1/2(receive new msg CAN1) -> [receive_CAN1_Sync_bc1_TAG]
  COMM Task - Sync BC1/3(send_new_msg_CAN2) -> [send_CAN2_Sync_bc1_TAG]
  [new_CAN2_msg_ready_TAG] -> COMM Task - Sync BC1/4(new_message_CAN2)
  [basic_cycle_TAG] -> COMM Task - Sync BC1/1(basic_cycle)
  COMM Task - Sync BC1/1(send_new_msg_CAN1) -> [send_CAN1_Sync_bc1_TAG]
  [local_ticks_TAG] -> COMM Task - Sync BC1/2(local_time)
  [new_CAN1_msg_ready_TAG] -> COMM Task - Sync BC1/3(new_message_CAN1)
  COMM Task - Sync BC1/4(receive_new_msg_CAN2) -> [receive_CAN2_Sync_bc1_TAG]
  [msg_Rx_TAG] -> COMP Task - Update LT - bc1/4(Rx_msg)
  [local_ticks_TAG] -> COMP Task - Update LT - bc1/2(local time)
  [new_msg_Rx_TAG] -> COMP Task - Update LT - bc1/3(new_message)
  [msg_Rx_CAN2_TAG] -> COMP Task - Rx_Sync_Check - bc1/6(Rx_msg_CAN2)
  [msg_Rx_CAN1_TAG] -> COMP Task - Rx_Sync_Check - bc1/5(Rx_msg_CAN1)
  [basic_cycle_TAG] -> COMP Task - Rx_Sync_Check - bc1/1(basic_cycle)
  [local_ticks_TAG] -> COMP Task - Rx_Sync_Check - bc1/2(local_time)
  [new_CAN2_msg_ready_TAG] -> COMP Task - Rx_Sync_Check - bc1/4(new_CAN2_msg)
  [new_CAN1_msg_ready_TAG] -> COMP Task - Rx_Sync_Check - bc1/3(new_CAN1_msg)
  [msg_Rx_TAG] -> COMP Task - Vote1 Count/4(Rx_msg)
  [msg_Rx_TAG] -> COMP Task - Vote2 Count/4(Rx_msg)
  [msg_Rx_TAG] -> COMP Task - Vote3 Count/4(Rx_msg)
  Data Store Read6/1 -> LT_Update Desync_Positive/Enable
  [local_ticks_TAG] -> LT_Update Desync_Positive/1(Local Time)

== system HANcoder_E407_GTSync_v5/HANcoder STM32 Target - E407-STM32 algorithm/Global Ticks Increment/CAN1 Recieve/Buffer ready ==
  note: CAN_Rx - Buffer
      | ready for new message
  note: Logic Analyzer - DEBUG
      | Rx Buffer Ready
  Enable : EnablePort
  Data Store Write : DataStoreWrite  DataStoreName=Rx_State_CAN1
  Data Store Write1 : DataStoreWrite  DataStoreName=Toggle_Pin_A0
  New_Msg : Constant  Value=2  OutDataTypeStr=uint8
  SET : Constant  OutDataTypeStr=boolean
  wires:
  New_Msg/1 -> Data Store Write/1
  SET/1 -> Data Store Write1/1

== system HANcoder_E407_GTSync_v5/HANcoder STM32 Target - E407-STM32 algorithm/Global Ticks Increment/CAN1 Recieve/CAN receive ==
  In1 : Inport
  Enabled Subsystem : Subsystem  TreatAsAtomicUnit=on
  S-Function : M-S-Function  FunctionName=sfcn_can_receive  Parameters=tsamp, canBus, outputNumber, dataType, byteOrder
  Out1 : Outport
  Out2 : Outport  Port=2
  Out3 : Outport  Port=3
  Out4 : Outport  Port=4
  Out5 : Outport  Port=5
  Out6 : Outport  Port=6
  Out7 : Outport  Port=7
  Out8 : Outport  Port=8
  Out9 : Outport  Port=9
  wires:
  S-Function/9 -> Enabled Subsystem/8(In8)
  S-Function/4 -> Enabled Subsystem/3(In3)
  S-Function/5 -> Enabled Subsystem/4(In4)
  S-Function/8 -> Enabled Subsystem/7(In7)
  S-Function/7 -> Enabled Subsystem/6(In6)
  S-Function/6 -> Enabled Subsystem/5(In5)
  Enabled Subsystem/8(Out8) -> Out9/1
  Enabled Subsystem/7(Out7) -> Out8/1
  Enabled Subsystem/6(Out6) -> Out7/1
  Enabled Subsystem/5(Out5) -> Out6/1
  Enabled Subsystem/4(Out4) -> Out5/1
  Enabled Subsystem/3(Out3) -> Out4/1
  Enabled Subsystem/2(Out2) -> Out3/1
  Enabled Subsystem/1(Out1) -> Out2/1
  S-Function/3 -> Enabled Subsystem/2(In2)
  S-Function/2 -> Enabled Subsystem/1(In1)
  S-Function/1 -> Out1/1, Enabled Subsystem/Enable
  In1/1 -> S-Function/1

== system HANcoder_E407_GTSync_v5/HANcoder STM32 Target - E407-STM32 algorithm/Global Ticks Increment/CAN1 Recieve/Prepare buffer ==
  note: Start preparing the buffer
  note: Logic Analyzer - DEBUG
      | Preparing Rx buffer
  Enable : EnablePort
  Constant1 : Constant  OutDataTypeStr=uint8
  Data Store Write : DataStoreWrite  DataStoreName=Rx_State_CAN1
  Data Store Write1 : DataStoreWrite  DataStoreName=Toggle_Pin_A0
  SET : Constant  OutDataTypeStr=boolean
  wires:
  Constant1/1 -> Data Store Write/1
  SET/1 -> Data Store Write1/1

== system HANcoder_E407_GTSync_v5/HANcoder STM32 Target - E407-STM32 algorithm/Global Ticks Increment/CAN1 Recieve/RxID_CAN ==
  RxID : Inport
  Bus Creator4 : BusCreator  Inputs=8
  Bus Selector : BusSelector  OutputSignals=signal1,signal2,signal3,signal4,signal5,signal6,signal7,signal8,signal9
  Bus Creator{,1..3} (4 alike) : BusCreator  Inputs=9
  Cast To Double{,1..3} (4 alike) : DataTypeConversion  OutDataTypeStr=double
  Constant : Constant  Value=Sync_ID
  Constant1 : Constant  Value=Vote1_ID
  Constant2 : Constant  Value=Vote2_ID
  Constant3 : Constant  Value=Vote3_ID
  Equal{,1..3} (4 alike) : RelationalOperator  Operator===  OutDataTypeStr=boolean  RndMeth=Simplest
  Switch : Switch  Criteria=u2 > Threshold
  Switch1 : Switch  Criteria=u2 > Threshold
  Switch2 : Switch  Criteria=u2 > Threshold
  Sync_ID_CAN : Subsystem
  Terminator{,1..3} (4 alike) : Terminator
  Vote1_ID_CAN : Subsystem
  Vote2_ID_CAN : Subsystem
  Vote3_ID_CAN : Subsystem
  CAN_new : Outport
  message : Outport  Port=2
  wires:
  Constant/1 -> Equal/2
  RxID/1 -> Equal2/1, Equal3/1, Equal1/1, Equal/1
  Equal/1 -> Sync_ID_CAN/Enable, Switch/2
  Constant1/1 -> Equal1/2
  Constant2/1 -> Equal2/2
  Constant3/1 -> Equal3/2
  Equal1/1 -> Vote1_ID_CAN/Enable, Switch1/2
  Equal2/1 -> Vote2_ID_CAN/Enable, Switch2/2
  Equal3/1 -> Vote3_ID_CAN/Enable
  Sync_ID_CAN/1(CAN_new) -> Bus Creator/1
  Sync_ID_CAN/2(Out2) -> Bus Creator/2
  Sync_ID_CAN/3(Out3) -> Bus Creator/3
  Sync_ID_CAN/4(Out4) -> Bus Creator/4
  Sync_ID_CAN/5(Out5) -> Bus Creator/5
  Sync_ID_CAN/6(Out6) -> Bus Creator/6
  Sync_ID_CAN/7(Out7) -> Bus Creator/7
  Sync_ID_CAN/8(Out8) -> Bus Creator/8
  Sync_ID_CAN/9(Out9) -> Bus Creator/9
  Bus Creator/1 -> Switch/1
  Vote1_ID_CAN/1(CAN_new) -> Bus Creator1/1
  Vote1_ID_CAN/2(Out2) -> Bus Creator1/2
  Vote1_ID_CAN/3(Out3) -> Bus Creator1/3
  Vote1_ID_CAN/4(Out4) -> Bus Creator1/4
  Vote1_ID_CAN/5(Out5) -> Bus Creator1/5
  Vote1_ID_CAN/6(Out6) -> Bus Creator1/6
  Vote1_ID_CAN/7(Out7) -> Bus Creator1/7
  Vote1_ID_CAN/8(Out8) -> Bus Creator1/8
  Vote1_ID_CAN/9(Out9) -> Bus Creator1/9
  Bus Creator1/1 -> Switch1/1
  Vote2_ID_CAN/1(CAN_new) -> Bus Creator2/1
  Vote2_ID_CAN/2(Out2) -> Bus Creator2/2
  Vote2_ID_CAN/3(Out3) -> Bus Creator2/3
  Vote2_ID_CAN/4(Out4) -> Bus Creator2/4
  Vote2_ID_CAN/6(Out6) -> Bus Creator2/6
  Vote2_ID_CAN/5(Out5) -> Bus Creator2/5
  Vote2_ID_CAN/7(Out7) -> Bus Creator2/7
  Vote2_ID_CAN/8(Out8) -> Bus Creator2/8
  Vote2_ID_CAN/9(Out9) -> Bus Creator2/9
  Bus Creator2/1 -> Switch2/1
  Vote3_ID_CAN/1(CAN_new) -> Bus Creator3/1
  Vote3_ID_CAN/2(Out2) -> Bus Creator3/2
  Vote3_ID_CAN/3(Out3) -> Bus Creator3/3
  Vote3_ID_CAN/4(Out4) -> Bus Creator3/4
  Vote3_ID_CAN/5(Out5) -> Bus Creator3/5
  Vote3_ID_CAN/6(Out6) -> Bus Creator3/6
  Vote3_ID_CAN/7(Out7) -> Bus Creator3/7
  Vote3_ID_CAN/8(Out8) -> Bus Creator3/8
  Vote3_ID_CAN/9(Out9) -> Bus Creator3/9
  Bus Creator3/1 -> Switch2/3
  Switch1/1 -> Switch/3
  Switch2/1 -> Switch1/3
  Switch/1 -> Bus Selector/1
  Bus Selector/1 -> CAN_new/1  "<signal1>"
  Bus Creator4/1 -> message/1
  Bus Selector/2 -> Bus Creator4/1, Cast To Double/1  "<signal2>"
  Bus Selector/6 -> Bus Creator4/5  "<signal6>"
  Bus Selector/7 -> Bus Creator4/6  "<signal7>"
  Bus Selector/8 -> Bus Creator4/7  "<signal8>"
  Bus Selector/9 -> Bus Creator4/8  "<signal9>"
  Cast To Double/1 -> Terminator/1  "RX_HDR_CAN1_s"
  Cast To Double1/1 -> Terminator1/1  "RX_LT1_CAN1_s"
  Bus Selector/3 -> Cast To Double1/1, Bus Creator4/2  "<signal3>"
  Bus Selector/4 -> Cast To Double2/1, Bus Creator4/3  "<signal4>"
  Cast To Double2/1 -> Terminator2/1  "RX_LT2_CAN1_s"
  Cast To Double3/1 -> Terminator3/1  "RX_BC_CAN1_s"
  Bus Selector/5 -> Cast To Double3/1, Bus Creator4/4  "<signal5>"

== system HANcoder_E407_GTSync_v5/HANcoder STM32 Target - E407-STM32 algorithm/Global Ticks Increment/CAN1 Recieve/Update message buffers ==
  note: Local time when the
      | message is received
  note: Received message
      | ready for processing
  note: CAN_Rx stop listening
  note: Logic Analyzer - DEBUG
      | Message received!
  message : Inport  OutDataTypeStr=Bus: msg_buffer_type
  Enable : EnablePort
  Bus Selector : BusSelector  OutputSignals=signal2,signal3,signal4,signal5,signal6,signal7,signal8,signal9
  Data Store Write : DataStoreWrite  DataStoreName=Toggle_Pin_A0
  Data Store Write1 : DataStoreWrite  DataStoreName=Msg_Rx_CAN1  DataStoreElements=Msg_Rx_CAN1.Buffer_1#Msg_Rx_CAN1.Buffer_2#Msg_Rx_CAN1.Buffer_3#Msg_Rx_CAN1.Buffer_4#Msg_Rx_CAN1.Buffer_5#Msg_Rx_CAN1.Buffer_6#Msg_Rx_CAN1.Buffer_7#Msg_Rx_CAN1.Buffer_8
  Data Store Write2 : DataStoreWrite  DataStoreName=New_Msg_Ready_CAN1
  Data Store Write5 : DataStoreWrite  DataStoreName=Rx_State_CAN1
  Data Store Write6 : DataStoreWrite  DataStoreName=Msg_Rx_Ticks_CAN1
  Idle_State : Constant  Value=3  OutDataTypeStr=uint8
  Local_Time : DataStoreRead  DataStoreName=Local_Ticks
  SET : Constant  OutDataTypeStr=boolean
  wires:
  Idle_State/1 -> Data Store Write5/1
  SET/1 -> Data Store Write/1, Data Store Write2/1
  Local_Time/1 -> Data Store Write6/1
  message/1 -> Bus Selector/1
  Bus Selector/1 -> Data Store Write1/1  "<signal2>"
  Bus Selector/2 -> Data Store Write1/2  "<signal3>"
  Bus Selector/3 -> Data Store Write1/3  "<signal4>"
  Bus Selector/4 -> Data Store Write1/4  "<signal5>"
  Bus Selector/5 -> Data Store Write1/5  "<signal6>"
  Bus Selector/6 -> Data Store Write1/6  "<signal7>"
  Bus Selector/7 -> Data Store Write1/7  "<signal8>"
  Bus Selector/8 -> Data Store Write1/8  "<signal9>"

== system HANcoder_E407_GTSync_v5/HANcoder STM32 Target - E407-STM32 algorithm/Global Ticks Increment/CAN1 Send/CAN send ==
  In1 : Inport
  In2 : Inport  Port=2
  In3 : Inport  Port=3
  In4 : Inport  Port=4
  In5 : Inport  Port=5
  In6 : Inport  Port=6
  In7 : Inport  Port=7
  In8 : Inport  Port=8
  In9 : Inport  Port=9
  S-Function : M-S-Function  FunctionName=sfcn_can_send  Parameters=tsamp, canBus, frameType, inputNumber, dataType, byteOrder
  wires:
  In1/1 -> S-Function/1
  In2/1 -> S-Function/2
  In3/1 -> S-Function/3
  In4/1 -> S-Function/4
  In5/1 -> S-Function/5
  In6/1 -> S-Function/6
  In7/1 -> S-Function/7
  In8/1 -> S-Function/8
  In9/1 -> S-Function/9

== system HANcoder_E407_GTSync_v5/HANcoder STM32 Target - E407-STM32 algorithm/Global Ticks Increment/CAN2 Recieve/Buffer ready ==
  note: Logic Analyzer - DEBUG
      | Rx Buffer Ready
  note: CAN_Rx - Buffer
      | ready for new message
  Enable : EnablePort
  Data Store Write : DataStoreWrite  DataStoreName=Rx_State_CAN2
  Data Store Write1 : DataStoreWrite  DataStoreName=Toggle_Pin_A0
  New_Msg : Constant  Value=2  OutDataTypeStr=uint8
  SET : Constant  OutDataTypeStr=boolean
  wires:
  SET/1 -> Data Store Write1/1
  New_Msg/1 -> Data Store Write/1

== system HANcoder_E407_GTSync_v5/HANcoder STM32 Target - E407-STM32 algorithm/Global Ticks Increment/CAN2 Recieve/CAN receive ==
  In1 : Inport
  Enabled Subsystem : Subsystem  TreatAsAtomicUnit=on
  S-Function : M-S-Function  FunctionName=sfcn_can_receive  Parameters=tsamp, canBus, outputNumber, dataType, byteOrder
  Out1 : Outport
  Out2 : Outport  Port=2
  Out3 : Outport  Port=3
  Out4 : Outport  Port=4
  Out5 : Outport  Port=5
  Out6 : Outport  Port=6
  Out7 : Outport  Port=7
  Out8 : Outport  Port=8
  Out9 : Outport  Port=9
  wires:
  S-Function/9 -> Enabled Subsystem/8(In8)
  S-Function/4 -> Enabled Subsystem/3(In3)
  S-Function/5 -> Enabled Subsystem/4(In4)
  S-Function/8 -> Enabled Subsystem/7(In7)
  S-Function/7 -> Enabled Subsystem/6(In6)
  S-Function/6 -> Enabled Subsystem/5(In5)
  Enabled Subsystem/8(Out8) -> Out9/1
  Enabled Subsystem/7(Out7) -> Out8/1
  Enabled Subsystem/6(Out6) -> Out7/1
  Enabled Subsystem/5(Out5) -> Out6/1
  Enabled Subsystem/4(Out4) -> Out5/1
  Enabled Subsystem/3(Out3) -> Out4/1
  Enabled Subsystem/2(Out2) -> Out3/1
  Enabled Subsystem/1(Out1) -> Out2/1
  S-Function/3 -> Enabled Subsystem/2(In2)
  S-Function/2 -> Enabled Subsystem/1(In1)
  S-Function/1 -> Out1/1, Enabled Subsystem/Enable
  In1/1 -> S-Function/1

== system HANcoder_E407_GTSync_v5/HANcoder STM32 Target - E407-STM32 algorithm/Global Ticks Increment/CAN2 Recieve/Prepare buffer ==
  note: Logic Analyzer - DEBUG
      | Preparing Rx buffer
  note: Start preparing the buffer
  Enable : EnablePort
  Constant1 : Constant  OutDataTypeStr=uint8
  Data Store Write : DataStoreWrite  DataStoreName=Rx_State_CAN2
  Data Store Write1 : DataStoreWrite  DataStoreName=Toggle_Pin_A0
  SET : Constant  OutDataTypeStr=boolean
  wires:
  SET/1 -> Data Store Write1/1
  Constant1/1 -> Data Store Write/1

== system HANcoder_E407_GTSync_v5/HANcoder STM32 Target - E407-STM32 algorithm/Global Ticks Increment/CAN2 Recieve/RxID_CAN ==
  RxID : Inport
  Bus Creator4 : BusCreator  Inputs=8
  Bus Selector : BusSelector  OutputSignals=signal1,signal2,signal3,signal4,signal5,signal6,signal7,signal8,signal9
  Bus Creator{,1..3} (4 alike) : BusCreator  Inputs=9
  Constant : Constant  Value=Sync_ID
  Constant1 : Constant  Value=Vote1_ID
  Constant2 : Constant  Value=Vote2_ID
  Constant3 : Constant  Value=Vote3_ID
  Equal{,1..3} (4 alike) : RelationalOperator  Operator===  OutDataTypeStr=boolean  RndMeth=Simplest
  Switch : Switch  Criteria=u2 > Threshold
  Switch1 : Switch  Criteria=u2 > Threshold
  Switch2 : Switch  Criteria=u2 > Threshold
  Sync_ID_CAN : Subsystem
  Vote1_ID_CAN : Subsystem
  Vote2_ID_CAN : Subsystem
  Vote3_ID_CAN : Subsystem
  CAN_new : Outport
  message : Outport  Port=2
  wires:
  Bus Selector/9 -> Bus Creator4/8  "<signal9>"
  Bus Selector/8 -> Bus Creator4/7  "<signal8>"
  Bus Selector/7 -> Bus Creator4/6  "<signal7>"
  Bus Selector/6 -> Bus Creator4/5  "<signal6>"
  Bus Selector/5 -> Bus Creator4/4  "<signal5>"
  Bus Selector/4 -> Bus Creator4/3  "<signal4>"
  Bus Selector/3 -> Bus Creator4/2  "<signal3>"
  Bus Selector/2 -> Bus Creator4/1  "<signal2>"
  Bus Creator4/1 -> message/1
  Bus Selector/1 -> CAN_new/1  "<signal1>"
  Switch/1 -> Bus Selector/1
  Switch2/1 -> Switch1/3
  Switch1/1 -> Switch/3
  Bus Creator3/1 -> Switch2/3
  Vote3_ID_CAN/9(Out9) -> Bus Creator3/9
  Vote3_ID_CAN/8(Out8) -> Bus Creator3/8
  Vote3_ID_CAN/7(Out7) -> Bus Creator3/7
  Vote3_ID_CAN/6(Out6) -> Bus Creator3/6
  Vote3_ID_CAN/5(Out5) -> Bus Creator3/5
  Vote3_ID_CAN/4(Out4) -> Bus Creator3/4
  Vote3_ID_CAN/3(Out3) -> Bus Creator3/3
  Vote3_ID_CAN/2(Out2) -> Bus Creator3/2
  Vote3_ID_CAN/1(CAN_new) -> Bus Creator3/1
  Bus Creator2/1 -> Switch2/1
  Vote2_ID_CAN/9(Out9) -> Bus Creator2/9
  Vote2_ID_CAN/8(Out8) -> Bus Creator2/8
  Vote2_ID_CAN/7(Out7) -> Bus Creator2/7
  Vote2_ID_CAN/5(Out5) -> Bus Creator2/5
  Vote2_ID_CAN/6(Out6) -> Bus Creator2/6
  Vote2_ID_CAN/4(Out4) -> Bus Creator2/4
  Vote2_ID_CAN/3(Out3) -> Bus Creator2/3
  Vote2_ID_CAN/2(Out2) -> Bus Creator2/2
  Vote2_ID_CAN/1(CAN_new) -> Bus Creator2/1
  Bus Creator1/1 -> Switch1/1
  Vote1_ID_CAN/9(Out9) -> Bus Creator1/9
  Vote1_ID_CAN/8(Out8) -> Bus Creator1/8
  Vote1_ID_CAN/7(Out7) -> Bus Creator1/7
  Vote1_ID_CAN/6(Out6) -> Bus Creator1/6
  Vote1_ID_CAN/5(Out5) -> Bus Creator1/5
  Vote1_ID_CAN/4(Out4) -> Bus Creator1/4
  Vote1_ID_CAN/3(Out3) -> Bus Creator1/3
  Vote1_ID_CAN/2(Out2) -> Bus Creator1/2
  Vote1_ID_CAN/1(CAN_new) -> Bus Creator1/1
  Bus Creator/1 -> Switch/1
  Sync_ID_CAN/9(Out9) -> Bus Creator/9
  Sync_ID_CAN/8(Out8) -> Bus Creator/8
  Sync_ID_CAN/7(Out7) -> Bus Creator/7
  Sync_ID_CAN/6(Out6) -> Bus Creator/6
  Sync_ID_CAN/5(Out5) -> Bus Creator/5
  Sync_ID_CAN/4(Out4) -> Bus Creator/4
  Sync_ID_CAN/3(Out3) -> Bus Creator/3
  Sync_ID_CAN/2(Out2) -> Bus Creator/2
  Sync_ID_CAN/1(CAN_new) -> Bus Creator/1
  Equal3/1 -> Vote3_ID_CAN/Enable
  Equal2/1 -> Switch2/2, Vote2_ID_CAN/Enable
  Equal1/1 -> Switch1/2, Vote1_ID_CAN/Enable
  Constant3/1 -> Equal3/2
  Constant2/1 -> Equal2/2
  Constant1/1 -> Equal1/2
  Equal/1 -> Switch/2, Sync_ID_CAN/Enable
  RxID/1 -> Equal/1, Equal1/1, Equal3/1, Equal2/1
  Constant/1 -> Equal/2

== system HANcoder_E407_GTSync_v5/HANcoder STM32 Target - E407-STM32 algorithm/Global Ticks Increment/CAN2 Recieve/Update message buffers ==
  note: Logic Analyzer - DEBUG
      | Message received!
  note: CAN_Rx stop listening
  note: Received message
      | ready for processing
  note: Local time when the
      | message is received
  message : Inport  OutDataTypeStr=Bus: msg_buffer_type
  Enable : EnablePort
  Bus Selector : BusSelector  OutputSignals=signal2,signal3,signal4,signal5,signal6,signal7,signal8,signal9
  Data Store Write : DataStoreWrite  DataStoreName=Toggle_Pin_A0
  Data Store Write1 : DataStoreWrite  DataStoreName=Msg_Rx_CAN2  DataStoreElements=Msg_Rx_CAN2.Buffer_1#Msg_Rx_CAN2.Buffer_2#Msg_Rx_CAN2.Buffer_3#Msg_Rx_CAN2.Buffer_4#Msg_Rx_CAN2.Buffer_5#Msg_Rx_CAN2.Buffer_6#Msg_Rx_CAN2.Buffer_7#Msg_Rx_CAN2.Buffer_8
  Data Store Write2 : DataStoreWrite  DataStoreName=New_Msg_Ready_CAN2
  Data Store Write5 : DataStoreWrite  DataStoreName=Rx_State_CAN2
  Data Store Write6 : DataStoreWrite  DataStoreName=Msg_Rx_Ticks_CAN2
  Idle_State : Constant  Value=3  OutDataTypeStr=uint8
  Local_Time : DataStoreRead  DataStoreName=Local_Ticks
  SET : Constant  OutDataTypeStr=boolean
  wires:
  Local_Time/1 -> Data Store Write6/1
  SET/1 -> Data Store Write2/1, Data Store Write/1
  message/1 -> Bus Selector/1
  Idle_State/1 -> Data Store Write5/1
  Bus Selector/1 -> Data Store Write1/1  "<signal2>"
  Bus Selector/2 -> Data Store Write1/2  "<signal3>"
  Bus Selector/3 -> Data Store Write1/3  "<signal4>"
  Bus Selector/4 -> Data Store Write1/4  "<signal5>"
  Bus Selector/5 -> Data Store Write1/5  "<signal6>"
  Bus Selector/6 -> Data Store Write1/6  "<signal7>"
  Bus Selector/7 -> Data Store Write1/7  "<signal8>"
  Bus Selector/8 -> Data Store Write1/8  "<signal9>"

== system HANcoder_E407_GTSync_v5/HANcoder STM32 Target - E407-STM32 algorithm/Global Ticks Increment/CAN2 Send/CAN send ==
  In1 : Inport
  In2 : Inport  Port=2
  In3 : Inport  Port=3
  In4 : Inport  Port=4
  In5 : Inport  Port=5
  In6 : Inport  Port=6
  In7 : Inport  Port=7
  In8 : Inport  Port=8
  In9 : Inport  Port=9
  S-Function : M-S-Function  FunctionName=sfcn_can_send  Parameters=tsamp, canBus, frameType, inputNumber, dataType, byteOrder
  wires:
  In9/1 -> S-Function/9
  In8/1 -> S-Function/8
  In7/1 -> S-Function/7
  In6/1 -> S-Function/6
  In5/1 -> S-Function/5
  In4/1 -> S-Function/4
  In3/1 -> S-Function/3
  In2/1 -> S-Function/2
  In1/1 -> S-Function/1

== system HANcoder_E407_GTSync_v5/HANcoder STM32 Target - E407-STM32 algorithm/Global Ticks Increment/Measure EXecution time/DEBUG - Toggle digital pin A3 ==
  note: Change pin state
  note: Toggle pin data stored
  Enable : EnablePort
  Constant : Constant  OutDataTypeStr=boolean
  Constant1 : Constant  Value=0  OutDataTypeStr=boolean
  Data Store Read : DataStoreRead  DataStoreName=A3_Pin_State
  Data Store Read1 : DataStoreRead  DataStoreName=A3_Pin_State
  Data Store Write1 : DataStoreWrite  DataStoreName=A3_Pin_State
  Digital Output : HANcoder_STM32_Target/STM32-E407/Digital Outputs/Digital Output  Tag=HANcoder_TARGET_STM32_E407  pinID=CON2 - A3  config=Open drain  tsamp=-1
      settings: SourceProductName=HANcoder STM32 Target
  Switch : Switch  Criteria=u2 > Threshold
  wires:
  Switch/1 -> Data Store Write1/1
  Data Store Read/1 -> Switch/2
  Constant/1 -> Switch/3
  Constant1/1 -> Switch/1
  Data Store Read1/1 -> Digital Output/1

== system HANcoder_E407_GTSync_v5/HANcoder STM32 Target - E407-STM32 algorithm/Global Ticks Increment/CAN Management/Initialization/Delay ==
  note: Update counter
      | < +1 tick every activation >
  note: Reset local counter
      | < for next activation >
  note: End of Delay
  Input : Inport
  Add2 : Sum
  Data Store Read : DataStoreRead  DataStoreName=Delay_Counter
  Data Store Read1 : DataStoreRead  DataStoreName=Delay_Counter
  Data Store Write2 : DataStoreWrite  DataStoreName=Delay_Counter
  GreaterThan : RelationalOperator  OutDataTypeStr=boolean  RndMeth=Simplest
  Increment1 : Constant  OutDataTypeStr=double
  Initializaton_Observation_DEBUG : Subsystem
  Reset : Constant  Value=-1  OutDataTypeStr=double
  Switch : Switch  Criteria=u2 > Threshold
  Output : Outport
  wires:
  Data Store Read/1 -> Add2/1
  Increment1/1 -> Add2/2
  Data Store Read1/1 -> GreaterThan/1
  Input/1 -> GreaterThan/2
  GreaterThan/1 -> Switch/2, Output/1
  Add2/1 -> Switch/3
  Reset/1 -> Switch/1
  Switch/1 -> Data Store Write2/1
